simulink model "pv2018_slx"  (R2018a)
settings: Solver=ode23tb  StartTime=0.0  StopTime=10  RelTol=1e-3  AbsTol=1e-3  EnableMultiTasking=on
libraries: powerlib x5, simulink x2
settings Model: Creator=Zekeriya_karaoglu  LastModifiedBy=Tolga
settings SolverCC: AutoScaleAbsTol=off
settings DataIOCC: LimitDataPoints=on  MaxDataPoints=10000
settings OptimizationCC: LifeSpan=inf
settings DebuggingCC: AllowSymbolicDim=off  SFUnexpectedBacktrackingDiag=warning  SFNoUnconditionalDefaultTransitionDiag=warning  SFExecutionAtInitializationDiag=none
settings CodeAppCC: StateflowObjectComments=on
settings GRTTargetCC: TargetLangStandard=C89/C90 (ANSI)  GeneratePreprocessorConditionals=Disable all
settings ConfigComp: CovMetricSettings=dw  CovHtmlReporting=on  CovSaveCumulativeToWorkspaceVar=on  CovSaveSingleToWorkspaceVar=on  CovExternalEMLEnable=off  CovSFcnEnable=off
settings SimscapeCC: SimscapeLogType=all  SimscapeLogDataHistory=10000

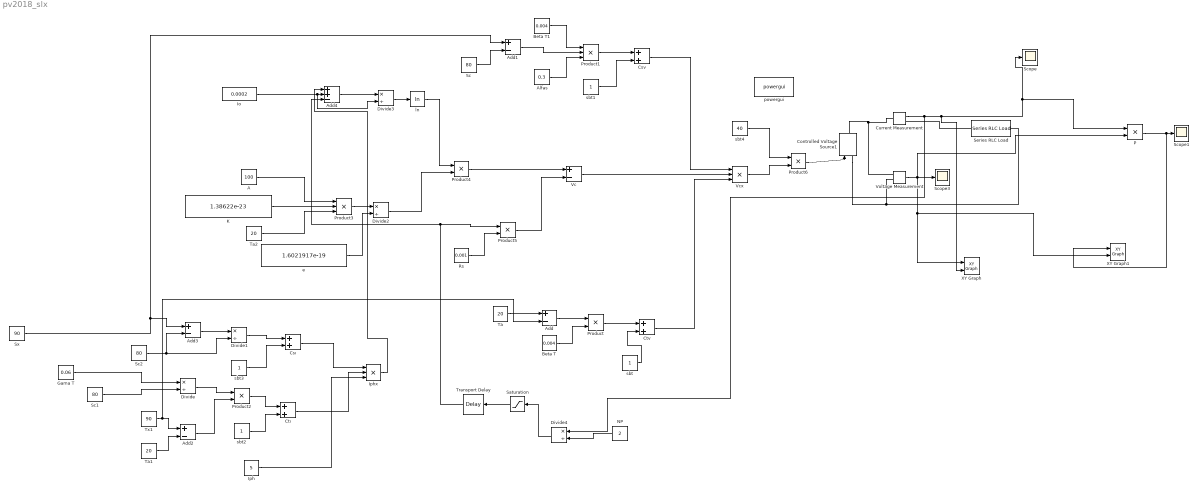
== system pv2018_slx ==
  A : Constant  Value=100
  Add{,1..3} (4 alike) : Sum  Inputs=+-
  Add4 : Sum  Inputs=++-
  "Alfas " : Constant  Value=0.3
  Beta T : Constant  Value=0.004
  Beta T1 : Constant  Value=0.004
  Controlled Voltage Source1 : powerlib/Electrical Sources/Controlled Voltage Source  Initialize=on  Source_Type=DC  Amplitude=100  Phase=0  Frequency=0  Measurements=None
  Csv : Sum
  Csı : Sum
  Ctv : Sum
  Ctı : Sum
  Current Measurement : powerlib/Measurements/Current Measurement  PhasorSimulation=off  OutputType=Complex  PSBequivalent=0
  Divide{,1..4} (5 alike) : Product  Inputs=*/
  Gama T : Constant  Value=0.06
  Io : Constant  Value=0.0002
  Iph : Constant  Value=5
  Iphx : Product  Inputs=3
  K : Constant  Value=1.38622e-23
  NP : Constant  Value=2
  P : Product
  Product{,2,4..6} (5 alike) : Product
  Product1 : Product  Inputs=3
  Product3 : Product  Inputs=3
  Rs : Constant  Value=0.001
  Saturation : Saturate  UpperLimit=inf  LowerLimit=-100  ZeroCross=off
  Sc : Constant  Value=80
  Sc1 : Constant  Value=80
  Sc2 : Constant  Value=80
  Scope : Scope
  Scope1 : Scope
  Scope3 : Scope
  Series RLC Load : powerlib/Elements/Series RLC Load  LConnTagsString=a  RConnTagsString=__new0  NominalVoltage=100  NominalFrequency=60  ActivePower=1000  InductivePower=0  CapacitivePower=0  Setx0=off  InitialVoltage=0  SetiL0=off  InitialCurrent=0  Measurements=None  LoadType=constant Z
  Sx : Constant  Value=90
  Ta : Constant  Value=20
  Ta1 : Constant  Value=20
  Ta2 : Constant  Value=20
  Transport Delay : TransportDelay  DelayTime=0.0001
  Tx1 : Constant  Value=90
  Vc : Sum  Inputs=+-
  Vcx : Product  Inputs=3
  Voltage Measurement : powerlib/Measurements/Voltage Measurement  PhasorSimulation=off  OutputType=Complex  PSBequivalent=0
  XY Graph : simulink/Sinks/XY Graph  xmin=47  xmax=53  ymin=4  ymax=6  st=50e-5
  XY Graph1 : simulink/Sinks/XY Graph  xmin=238  xmax=280  ymin=49  ymax=54  st=50e-5
  e : Constant  Value=1.6021917e-19
  ln : Math  Operator=log  SaturateOnIntegerOverflow=on
  powergui : powerlib/powergui  Priority=1  SimulationMode=Discrete  SampleTime=50e-5  frequency=60  Iterations=50  frequencyindice=0  Pbase=100e6  ErrMax=1e-4  UnitsV=kV  UnitsW=MW  buscounter=0  FunctionMessages=off  echomessages=off  EnableUseOfTLC=off  CurrentSourceSwitches=off  DisableSnubberDevices=off  DisableRonSwitches=off  DisableVfSwitches=off  DisplayEquations=off  SolverType=Tustin/Backward Euler (TBE)  Interpol=off  ExternalGateDelay=off  methode=off  Ts=100  x0status=blocks  SPID=on  SwTol=0  HookPort=off  RestoreLinks=warning  ResistiveCurrentMeasurement=off  Frange=[0:2:500]  Ylog=off  Xlog=on  ShowGrid=off  save=off  variable=ZData  structure=0  ZoomFFT=off  StartTime=0.0  cycles=1  DisplayStyle=1  fundamental=60  FreqAxis=off  MaxFrequency=1000  frequencyindicesteady=1  RmsSteady=1  display=off
  sbt{,1..3} (4 alike) : Constant
  sbt4 : Constant  Value=40
  wires:
  Rs/1 -> Product5/2
  Csı/1 -> Iphx/1
  Divide2/1 -> Product4/2
  Iph/1 -> Iphx/3
  Io/1 -> Divide3/2, Add4/2
  ln/1 -> Product4/1
  Vc/1 -> Vcx/2
  Divide3/1 -> ln/1
  Ta/1 -> Add/1
  Add1/1 -> Product1/2
  Ta2/1 -> Product3/3
  Ctv/1 -> Vcx/3
  Sx/1 -> Add1/1, Add3/1
  Add/1 -> Product/1
  sbt3/1 -> Csı/2
  Product4/1 -> Vc/1
  Ctı/1 -> Iphx/2
  e/1 -> Divide2/2
  Product2/1 -> Ctı/1
  Sc2/1 -> Divide1/2, Add3/2
  Add3/1 -> Divide1/1
  Gama T/1 -> Divide/1
  Add2/1 -> Product2/2
  Product3/1 -> Divide2/1
  Add4/1 -> Divide3/1
  sbt1/1 -> Csv/2
  Divide1/1 -> Csı/1
  Ta1/1 -> Add2/2
  Divide/1 -> Product2/1
  Beta T/1 -> Product/2
  Product1/1 -> Csv/1
  sbt2/1 -> Ctı/2
  "Alfas "/1 -> Product1/3
  Beta T1/1 -> Product1/1
  sbt/1 -> Ctv/2
  Sc1/1 -> Divide/2
  Csv/1 -> Vcx/1
  Product5/1 -> Vc/2
  Tx1/1 -> Add/2, Add2/1
  Product/1 -> Ctv/1
  K/1 -> Product3/2
  A/1 -> Product3/1
  Sc/1 -> Add1/2
  Saturation/1 -> Transport Delay/1
  Transport Delay/1 -> Add4/3, Product5/1
  Iphx/1 -> Add4/1
  Vcx/1 -> Product6/2
  Product6/1 -> Controlled Voltage Source1/1
  sbt4/1 -> Product6/1
  Current Measurement/1 -> Divide4/1, XY Graph/2, P/1, Scope/1
  NP/1 -> Divide4/2
  Divide4/1 -> Saturation/1
  Voltage Measurement/1 -> P/2, XY Graph1/2, XY Graph/1, Scope3/1
  P/1 -> XY Graph1/1, Scope1/1
  connections:
  Voltage Measurement/LConn1 -- Current Measurement/LConn1 -- Controlled Voltage Source1/RConn1
  Series RLC Load/LConn1 -- Current Measurement/RConn1
  Voltage Measurement/LConn2 -- Controlled Voltage Source1/LConn1 -- Series RLC Load/RConn1
